simulink model "WESDem_SetPoint"  (R2016b)
settings: configuration reference "CodeGenConfigSet" (kept outside this file)
values from neighbouring files (symbols this model uses):
  EISGov_st3valid_C = Calibration.Parameter    [init_WESDem_SetPoint.m]
  WESDem_dnAcc0_C = Calibration.Parameter    [init_WESDem_SetPoint.m]
  WESDem_dnAcc1_C = Calibration.Parameter    [init_WESDem_SetPoint.m]
  WESDem_dnAcc3_C = Calibration.Parameter    [init_WESDem_SetPoint.m]
  WESDem_dnDecn0_C = Calibration.Parameter    [init_WESDem_SetPoint.m]
  WESDem_dnDecn1_C = Calibration.Parameter    [init_WESDem_SetPoint.m]
  WESDem_dnDecn2_C = Calibration.Parameter    [init_WESDem_SetPoint.m]
  WESDem_nDelta_C = Calibration.Parameter    [init_WESDem_SetPoint.m]
  WESDem_nMin0_C = Calibration.Parameter    [init_WESDem_SetPoint.m]
  WESDem_nMin1_C = Calibration.Parameter    [init_WESDem_SetPoint.m]
  WESDem_nMin2_C = Calibration.Parameter    [init_WESDem_SetPoint.m]
  WESDem_nMin3_C = Calibration.Parameter    [init_WESDem_SetPoint.m]
  WESDem_nMode0_C = Calibration.Parameter    [init_WESDem_SetPoint.m]
  WESDem_nMode1_C = Calibration.Parameter    [init_WESDem_SetPoint.m]
  WESDem_nMode2_C = Calibration.Parameter    [init_WESDem_SetPoint.m]
  WESDem_nMode3_C = Calibration.Parameter    [init_WESDem_SetPoint.m]
  WESDem_nSetPHi0_C = Calibration.Parameter    [init_WESDem_SetPoint.m]
  WESDem_nSetPHi1_C = Calibration.Parameter    [init_WESDem_SetPoint.m]
  WESDem_nSetPHi2_C = Calibration.Parameter    [init_WESDem_SetPoint.m]
  WESDem_nSetPHi3_C = Calibration.Parameter    [init_WESDem_SetPoint.m]
  WESDem_nTipStp_C = Calibration.Parameter    [init_WESDem_SetPoint.m]
  WESDem_rAPPThresFrzI_C = Calibration.Parameter    [init_WESDem_SetPoint.m]
  WESDem_SetPLoTipInRmpSlopeNeg_C = Calibration.Parameter    [init_WESDem_SetPoint.m]
  WESDem_SetPLoTipInRmpSlopePos_C = Calibration.Parameter    [init_WESDem_SetPoint.m]
  WESDem_stASDrfInit_C = Calibration.Parameter    [init_WESDem_SetPoint.m]
  WESDem_stCurr_C = Calibration.Parameter    [init_WESDem_SetPoint.m]
  WESDem_stCurrvalid_C = Calibration.Parameter    [init_WESDem_SetPoint.m]
  WESDem_stMskFrzRls_C = Calibration.Parameter    [init_WESDem_SetPoint.m]
  WESDem_swtTrqHiSel_C = Calibration.Parameter    [init_WESDem_SetPoint.m]
  WESDem_swtTrqLoSel_C = Calibration.Parameter    [init_WESDem_SetPoint.m]
  WESDem_tiPT1_C = Calibration.Parameter    [init_WESDem_SetPoint.m]
  WESDem_tiTrqHiPT1_C = Calibration.Parameter    [init_WESDem_SetPoint.m]
  WESDem_tiTrqLoPT1_C = Calibration.Parameter    [init_WESDem_SetPoint.m]
undefined symbols (not defined in the file or in its folder): CruiseCtl_State_conv, Switch_conv, WESDem_SetPoint_DT, WESDem_State_conv
libraries: CXLib x23, simulink x15
(part 2 of 2)

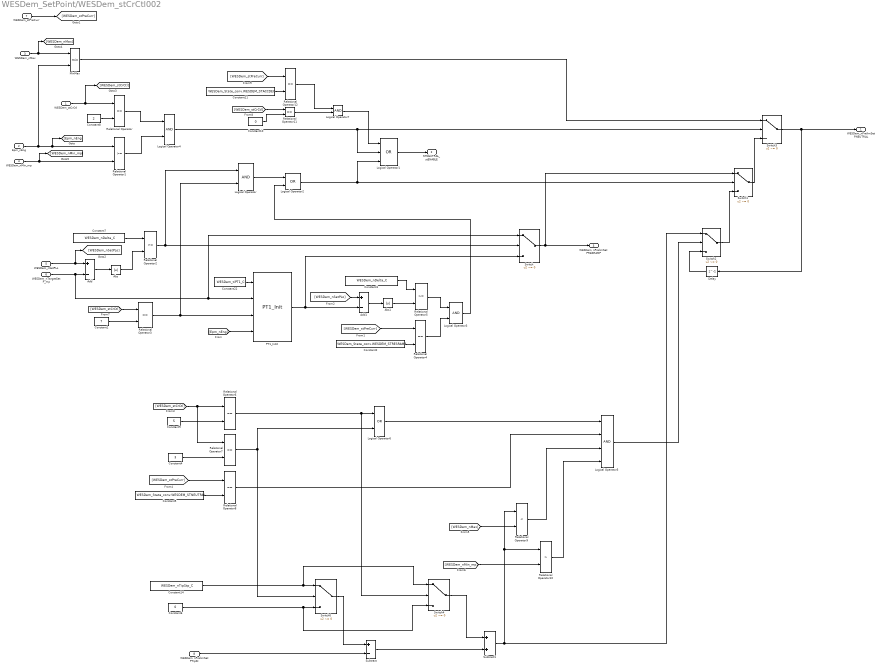
== system WESDem_SetPoint/WESDem_stCrCtl002  ==
  WESDem_stCrCtl : Inport  Description=State control of the working engine speed demand  OutMin=0  OutMax=65535  OutDataTypeStr=State_uint16
  Epm_nEng : Inport  Tag=rpm  Description=Engine speed  Port=2  OutMin=0  OutMax=6000  OutDataTypeStr=EngSpeed_rpm
  WESDem_nMax : Inport  Tag=rpm  Description=Engine speed  Port=3  OutMin=0  OutMax=6000  OutDataTypeStr=EngSpeed_rpm
  WESDem_nMin_mp : Inport  Tag=rpm  Description=Engine speed  Port=4  OutMin=0  OutMax=6000  OutDataTypeStr=EngSpeed_rpm
  WESDem_nSetPLo : Inport  Port=5
  WESDem_nTargetSetP_mp : Inport  Port=6
  WESDem_stPreCurr : Inport  Description=State control of the working engine speed demand  Port=7  OutDataTypeStr=Enum: WESDem_State_conv
  WESDem_nPrelimSetPTipSt : Inport  Port=8
  Abs : Abs
  Abs1 : Abs
  Add : Sum  Inputs=+-
  Add1 : Sum  Inputs=+-
  Constant1 : Constant  Value=7  OutDataTypeStr=Inherit: Inherit via back propagation
  Constant10 : Constant  Value=0  OutDataTypeStr=Inherit: Inherit via back propagation
  Constant11 : Constant  Value=WESDem_State_conv.WESDEM_STACCDEC  OutDataTypeStr=Inherit: Inherit via back propagation
  Constant14 : Constant  Value=WESDem_nTipStp_C
  Constant2 : Constant  Value=WESDem_State_conv.WESDEM_STRESRAMP  OutDataTypeStr=Inherit: Inherit via back propagation
  Constant22 : Constant  Value=WESDem_tiPT1_C
  Constant3 : Constant  Value=WESDem_nDelta_C
  Constant4 : Constant  Value=3  OutDataTypeStr=Inherit: Inherit via back propagation
  Constant5 : Constant  Value=WESDem_State_conv.WESDEM_STNEUTRAL  OutDataTypeStr=Inherit: Inherit via back propagation
  Constant6 : Constant  Value=0  OutDataTypeStr=Inherit: Inherit via back propagation
  Constant7 : Constant  Value=WESDem_nDelta_C
  Constant8 : Constant  Value=2  OutDataTypeStr=Inherit: Inherit via back propagation
  Constant9 : Constant  Value=5  OutDataTypeStr=Inherit: Inherit via back propagation
  Delay : Delay  DelayLength=1  InitialCondition=0
  Logical Operator{,3..4,7} (4 alike) : Logic  AllPortsSameDT=off  OutDataTypeStr=boolean
  Logical Operator1 : Logic  Operator=OR  Inputs=3  AllPortsSameDT=off  OutDataTypeStr=boolean
  Logical Operator2 : Logic  Operator=OR  AllPortsSameDT=off  OutDataTypeStr=boolean
  Logical Operator5 : Logic  Inputs=4  AllPortsSameDT=off  OutDataTypeStr=boolean
  Logical Operator6 : Logic  Operator=OR  AllPortsSameDT=off  OutDataTypeStr=boolean
  MinMax : MinMax  Inputs=2
  PT1_Init2 : CXLib/PT1_Init
  Relational Operator{,3..4,8,11..12} (6 alike) : RelationalOperator  Operator===  OutDataTypeStr=boolean  RndMeth=Simplest
  Relational Operator1 : RelationalOperator  OutDataTypeStr=boolean  RndMeth=Simplest
  Relational Operator10 : RelationalOperator  Operator=>  OutDataTypeStr=boolean  RndMeth=Simplest
  Relational Operator2 : RelationalOperator  OutDataTypeStr=boolean  RndMeth=Simplest
  Relational Operator5 : RelationalOperator  OutDataTypeStr=boolean  RndMeth=Simplest
  Relational Operator6 : RelationalOperator  Operator===  OutDataTypeStr=boolean  RndMeth=Simplest  InputSameDT=on
  Relational Operator7 : RelationalOperator  Operator===  OutDataTypeStr=boolean  RndMeth=Simplest  InputSameDT=on
  Relational Operator9 : RelationalOperator  Operator=<  OutDataTypeStr=boolean  RndMeth=Simplest
  Subtract : Sum  Inputs=+-
  Subtract1 : Sum
  Switch{,1..4,6} (6 alike) : Switch  Criteria=u2 ~= 0
  WESDem_nPrelimSetPNEUTRAL : Outport  Tag=rpm  Description=maximum engine speed in selected mode  OutMin=0  OutMax=6000  OutDataTypeStr=EngSpeed_rpm
  STNEUTRAL_stENABLE : Outport  Port=2
  WESDem_nPrelimSetPRESRAMP : Outport  Port=3
  wires:
  WESDem_stCrCtl/1 -> Relational Operator/1, [WESDem_stCrCtl]
  Constant8/1 -> Relational Operator/2
  Epm_nEng/1 -> MinMax/2, Relational Operator1/1, [Epm_nEng]
  WESDem_nMin_mp/1 -> Relational Operator1/2, [WESDem_nMin_mp]
  Relational Operator/1 -> Logical Operator4/1
  Relational Operator1/1 -> Logical Operator4/2
  WESDem_nMax/1 -> MinMax/1, [WESDem_nMax]
  MinMax/1 -> Switch3/1
  Logical Operator4/1 -> Logical Operator1/2, Switch3/2
  Switch3/1 -> Delay/1, WESDem_nPrelimSetPNEUTRAL/1
  Abs/1 -> Relational Operator2/2
  Constant7/1 -> Relational Operator2/1
  WESDem_nSetPLo/1 -> [WESDem_nSetPLo], Add/1
  Add/1 -> Abs/1
  WESDem_nTargetSetP_mp/1 -> Switch/1, PT1_Init2/2, Add/2
  Constant1/1 -> Relational Operator3/2
  Relational Operator2/1 -> Logical Operator/1, Switch/2
  Logical Operator1/1 -> STNEUTRAL_stENABLE/1
  WESDem_stPreCurr/1 -> [WESDem_stPreCurr]
  PT1_Init2/1 -> Switch/3, Add1/2
  Constant22/1 -> PT1_Init2/1
  Relational Operator3/1 -> Logical Operator/2, PT1_Init2/3
  [Epm_nEng] -> PT1_Init2/4
  Switch1/1 -> Switch3/3
  Switch/1 -> WESDem_nPrelimSetPRESRAMP/1, Switch1/1
  Logical Operator/1 -> Logical Operator2/1
  Constant2/1 -> Relational Operator4/2
  [WESDem_stPreCurr] -> Relational Operator4/1
  Add1/1 -> Abs1/1
  [WESDem_nSetPLo] -> Add1/1
  Constant3/1 -> Relational Operator5/1
  Abs1/1 -> Relational Operator5/2
  Relational Operator5/1 -> Logical Operator3/1
  Relational Operator4/1 -> Logical Operator3/2
  Logical Operator3/1 -> Logical Operator2/2
  Logical Operator2/1 -> Logical Operator1/3, Switch1/2
  Delay/1 -> Switch2/3
  [WESDem_stCrCtl] -> Relational Operator7/1, Relational Operator6/1
  Constant9/1 -> Relational Operator6/2
  Constant4/1 -> Relational Operator7/2
  Relational Operator7/1 -> Switch6/2, Logical Operator6/2
  Relational Operator6/1 -> Switch4/2, Logical Operator6/1
  [WESDem_stPreCurr] -> Relational Operator8/1
  Constant5/1 -> Relational Operator8/2
  Logical Operator6/1 -> Logical Operator5/1
  Relational Operator8/1 -> Logical Operator5/2
  [WESDem_nMax] -> Relational Operator9/2
  Relational Operator9/1 -> Logical Operator5/3
  [WESDem_nMin_mp] -> Relational Operator10/2
  Constant6/1 -> Switch4/3, Switch6/3
  Constant14/1 -> Switch4/1, Switch6/1
  WESDem_nPrelimSetPTipSt/1 -> Subtract/2
  Switch6/1 -> Subtract/1
  Switch4/1 -> Subtract1/1
  Subtract/1 -> Subtract1/2
  Relational Operator10/1 -> Logical Operator5/4
  Subtract1/1 -> Switch2/1, Relational Operator10/1, Relational Operator9/1
  Logical Operator5/1 -> Switch2/2
  Switch2/1 -> Switch1/3
  [WESDem_stCrCtl] -> Relational Operator3/1
  [WESDem_stCrCtl] -> Relational Operator11/1
  Constant10/1 -> Relational Operator11/2
  Relational Operator11/1 -> Logical Operator7/2
  Constant11/1 -> Relational Operator12/2
  [WESDem_stPreCurr] -> Relational Operator12/1
  Relational Operator12/1 -> Logical Operator7/1
  Logical Operator7/1 -> Logical Operator1/1

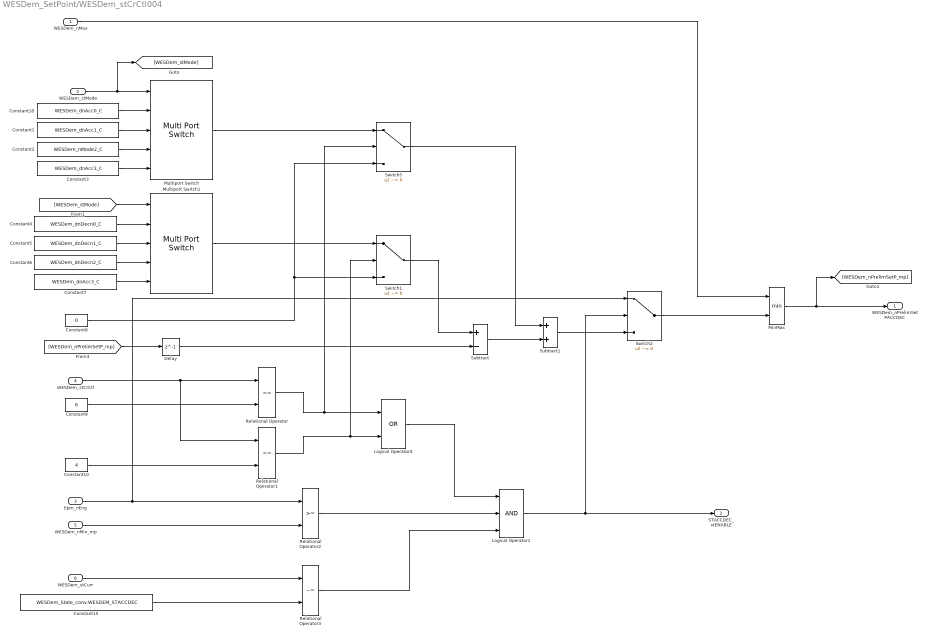
== system WESDem_SetPoint/WESDem_stCrCtl004 ==
  WESDem_nMax : Inport  Tag=rpm  Description=Working engine speed setpoint through start button  OutMin=0  OutMax=6000  OutDataTypeStr=EngSpeed_rpm
  WESDem_stMode : Inport  Description=Operating mode of the working engine speed demand  Port=2  OutMin=0  OutMax=255  OutDataTypeStr=State_uint8
  Epm_nEng : Inport  Tag=rpm  Description=Engine speed  Port=3  OutMin=0  OutMax=6000  OutDataTypeStr=EngSpeed_rpm
  WESDem_stCrCtl : Inport  Description=State control of the working engine speed demand  Port=4  OutMin=0  OutMax=65535  OutDataTypeStr=State_uint16
  WESDem_nMin_mp : Inport  Port=5
  WESDem_stCurr : Inport  Port=6
  Constant1 : Constant  Value=WESDem_dnAcc1_C
  Constant10 : Constant  Value=4
  Constant15 : Constant  Value=WESDem_State_conv.WESDEM_STACCDEC  OutDataTypeStr=Inherit: Inherit via back propagation
  Constant18 : Constant  Value=WESDem_dnAcc0_C
  Constant2 : Constant  Value=WESDem_nMode2_C
  Constant3 : Constant  Value=WESDem_dnAcc3_C
  Constant4 : Constant  Value=WESDem_dnDecn0_C
  Constant5 : Constant  Value=WESDem_dnDecn1_C
  Constant6 : Constant  Value=WESDem_dnDecn2_C
  Constant7 : Constant  Value=WESDem_dnAcc3_C
  Constant8 : Constant  Value=0  OutDataTypeStr=Inherit: Inherit via back propagation
  Constant9 : Constant  Value=6
  Delay : Delay  DelayLength=1  InitialCondition=0
  Logical Operator1 : Logic  Inputs=3  AllPortsSameDT=off  OutDataTypeStr=boolean
  Logical Operator4 : Logic  Operator=OR  AllPortsSameDT=off  OutDataTypeStr=boolean
  MinMax : MinMax  Inputs=2
  Multiport Switch : MultiPortSwitch  DataPortOrder=Zero-based contiguous  Inputs=4
  Multiport Switch1 : MultiPortSwitch  DataPortOrder=Zero-based contiguous  Inputs=4
  Relational Operator : RelationalOperator  Operator===  OutDataTypeStr=boolean  RndMeth=Simplest
  Relational Operator1 : RelationalOperator  Operator===  OutDataTypeStr=boolean  RndMeth=Simplest
  Relational Operator2 : RelationalOperator  OutDataTypeStr=boolean  RndMeth=Simplest
  Relational Operator3 : RelationalOperator  Operator=~=  OutDataTypeStr=boolean  RndMeth=Simplest
  Subtract : Sum  Inputs=+-
  Subtract1 : Sum
  Switch1 : Switch  Criteria=u2 ~= 0
  Switch2 : Switch  Criteria=u2 ~= 0
  Switch5 : Switch  Criteria=u2 ~= 0
  WESDem_nPrelimSetPACCDEC : Outport  Tag=rpm  Description=maximum engine speed in selected mode  OutMin=0  OutMax=6000  OutDataTypeStr=EngSpeed_rpm
  STACCDEC_stENABLE : Outport  Port=2
  wires:
  WESDem_stMode/1 -> [WESDem_stMode], Multiport Switch/1
  Constant1/1 -> Multiport Switch/3
  Constant2/1 -> Multiport Switch/4
  Constant3/1 -> Multiport Switch/5
  Constant18/1 -> Multiport Switch/2
  Constant4/1 -> Multiport Switch1/2
  Constant5/1 -> Multiport Switch1/3
  Constant6/1 -> Multiport Switch1/4
  Constant7/1 -> Multiport Switch1/5
  Multiport Switch/1 -> Switch5/1
  Multiport Switch1/1 -> Switch1/1
  Constant8/1 -> Switch1/3, Switch5/3
  Switch1/1 -> Subtract/1
  Delay/1 -> Subtract/2
  Switch5/1 -> Subtract1/1
  Subtract/1 -> Subtract1/2
  Subtract1/1 -> Switch2/3
  WESDem_stCrCtl/1 -> Relational Operator1/1, Relational Operator/1
  Constant9/1 -> Relational Operator/2
  Constant10/1 -> Relational Operator1/2
  Relational Operator/1 -> Switch5/2, Logical Operator4/1
  Relational Operator1/1 -> Switch1/2, Logical Operator4/2
  Epm_nEng/1 -> Switch2/1, Relational Operator2/1
  [WESDem_stMode] -> Multiport Switch1/1
  Constant15/1 -> Relational Operator3/2
  Relational Operator3/1 -> Logical Operator1/3
  Relational Operator2/1 -> Logical Operator1/2
  Logical Operator4/1 -> Logical Operator1/1
  Logical Operator1/1 -> Switch2/2, STACCDEC_stENABLE/1
  Switch2/1 -> MinMax/2
  WESDem_nMax/1 -> MinMax/1
  MinMax/1 -> [WESDem_nPrelimSetP_mp], WESDem_nPrelimSetPACCDEC/1
  [WESDem_nPrelimSetP_mp] -> Delay/1
  WESDem_nMin_mp/1 -> Relational Operator2/2
  WESDem_stCurr/1 -> Relational Operator3/1

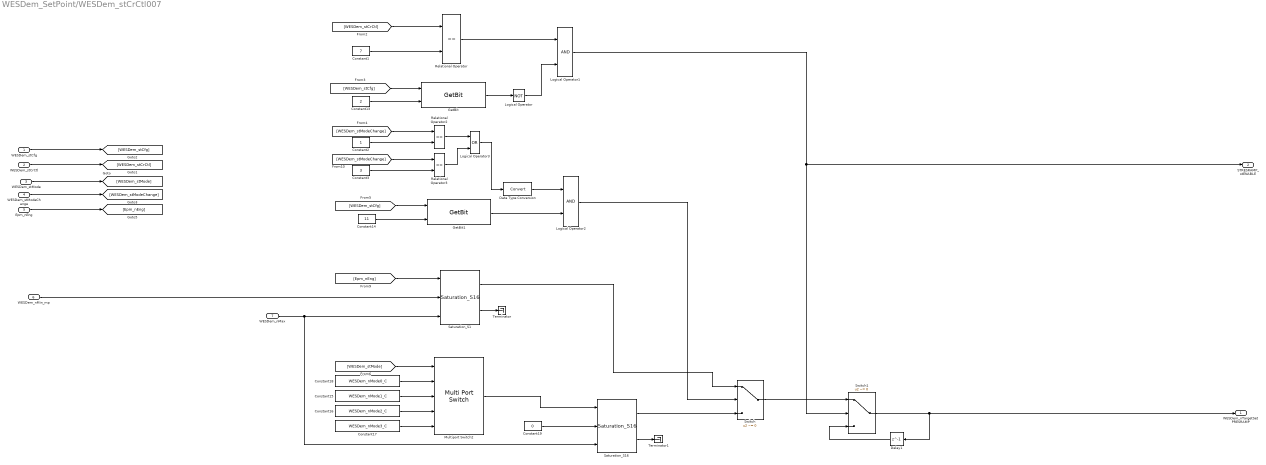
== system WESDem_SetPoint/WESDem_stCrCtl007 ==
  WESDem_stCfg : Inport  Description=Configuration of the actual operating mode  OutMin=0  OutMax=65535  OutDataTypeStr=State_uint16
  WESDem_stCrCtl : Inport  Description=State control of the working engine speed demand  Port=2  OutMin=0  OutMax=65535  OutDataTypeStr=State_uint16
  WESDem_stMode : Inport  Description=Operating mode of the working engine speed demand  Port=3  OutMin=0  OutMax=255  OutDataTypeStr=State_uint8
  WESDem_stModeChange : Inport  Description=Operating mode change of the working engine speed demand  Port=4  OutMin=0  OutMax=255  OutDataTypeStr=State_uint8
  Epm_nEng : Inport  Tag=rpm  Description=Engine speed  Port=5  OutMin=0  OutMax=6000  OutDataTypeStr=EngSpeed_rpm
  WESDem_nMin_mp : Inport  Port=6
  WESDem_nMax : Inport  Port=7
  Constant1 : Constant  Value=7  OutDataTypeStr=Inherit: Inherit via back propagation
  Constant13 : Constant  Value=2  OutDataTypeStr=Inherit: Inherit via back propagation
  Constant14 : Constant  Value=11  OutDataTypeStr=Inherit: Inherit via back propagation
  Constant15 : Constant  Value=WESDem_nMode1_C
  Constant16 : Constant  Value=WESDem_nMode2_C
  Constant17 : Constant  Value=WESDem_nMode3_C
  Constant18 : Constant  Value=WESDem_nMode0_C
  Constant19 : Constant  Value=0  OutDataTypeStr=Inherit: Inherit via back propagation
  Constant2 : Constant  OutDataTypeStr=Inherit: Inherit via back propagation
  Constant3 : Constant  Value=3  OutDataTypeStr=Inherit: Inherit via back propagation
  Data Type Conversion : DataTypeConversion
  Delay1 : Delay  DelayLength=1  InitialCondition=0
  GetBit : CXLib/GetBit  dataTypeString=uint16  dataLength=0
      settings: AttributesFormatString=Get bit from %<dataTypeString>
  GetBit1 : CXLib/GetBit  dataTypeString=uint16  dataLength=0
      settings: AttributesFormatString=Get bit from %<dataTypeString>
  Logical Operator : Logic  Operator=NOT  AllPortsSameDT=off  OutDataTypeStr=boolean
  Logical Operator1 : Logic  AllPortsSameDT=off  OutDataTypeStr=boolean
  Logical Operator2 : Logic  AllPortsSameDT=off  OutDataTypeStr=boolean
  Logical Operator3 : Logic  Operator=OR  AllPortsSameDT=off  OutDataTypeStr=boolean
  Multiport Switch2 : MultiPortSwitch  DataPortOrder=Zero-based contiguous  Inputs=4
  Relational Operator : RelationalOperator  Operator===  OutDataTypeStr=boolean  RndMeth=Simplest
  Relational Operator2 : RelationalOperator  Operator===  OutDataTypeStr=boolean  RndMeth=Simplest
  Relational Operator3 : RelationalOperator  Operator===  OutDataTypeStr=boolean  RndMeth=Simplest
  Saturation_S1 : CXLib/Saturation_S16
  Saturation_S16 : CXLib/Saturation_S16
  Switch : Switch  Criteria=u2 ~= 0
  Switch1 : Switch  Criteria=u2 ~= 0
  Terminator : Terminator
  Terminator1 : Terminator
  WESDem_nTargetSetPRESRAMP : Outport  Description=Status of the working engine Speed Control  OutMin=0  OutMax=6000  OutDataTypeStr=EngSpeed_rpm
  STRESRAMP_stENABLE : Outport  Port=2
  wires:
  Delay1/1 -> Switch1/3
  WESDem_stCrCtl/1 -> [WESDem_stCrCtl]
  WESDem_stMode/1 -> [WESDem_stMode]
  Relational Operator/1 -> Logical Operator1/1
  [WESDem_stCfg] -> GetBit1/1
  Epm_nEng/1 -> [Epm_nEng]
  Saturation_S1/1 -> Switch/1
  Constant14/1 -> GetBit1/2
  [Epm_nEng] -> Saturation_S1/1
  WESDem_stModeChange/1 -> [WESDem_stModeChange]
  Logical Operator/1 -> Logical Operator1/2
  Saturation_S16/1 -> Switch/3
  Multiport Switch2/1 -> Saturation_S16/1
  WESDem_nMax/1 -> Saturation_S16/3, Saturation_S1/3
  [WESDem_stMode] -> Multiport Switch2/1
  GetBit1/1 -> Logical Operator2/2
  Constant15/1 -> Multiport Switch2/3
  Logical Operator2/1 -> Switch/2
  Constant19/1 -> Saturation_S16/2
  WESDem_stCfg/1 -> [WESDem_stCfg]
  [WESDem_stCfg] -> GetBit/1
  Constant13/1 -> GetBit/2
  Constant1/1 -> Relational Operator/2
  Constant18/1 -> Multiport Switch2/2
  GetBit/1 -> Logical Operator/1
  Constant16/1 -> Multiport Switch2/4
  [WESDem_stCrCtl] -> Relational Operator/1
  Constant17/1 -> Multiport Switch2/5
  Saturation_S16/2 -> Terminator1/1
  Switch/1 -> Switch1/1
  Logical Operator1/1 -> STRESRAMP_stENABLE/1, Switch1/2
  Saturation_S1/2 -> Terminator/1
  Switch1/1 -> Delay1/1, WESDem_nTargetSetPRESRAMP/1
  Data Type Conversion/1 -> Logical Operator2/1
  [WESDem_stModeChange] -> Relational Operator2/1
  Constant2/1 -> Relational Operator2/2
  [WESDem_stModeChange] -> Relational Operator3/1
  Constant3/1 -> Relational Operator3/2
  Relational Operator2/1 -> Logical Operator3/1
  Relational Operator3/1 -> Logical Operator3/2
  Logical Operator3/1 -> Data Type Conversion/1
  WESDem_nMin_mp/1 -> Saturation_S1/2

== stateflow chart WESDem_SetPoint/EISGov initialization/Chart ==
  state WESDEM_STNOINIT
    entry:WESDem_stEISGovInit_mp = 0;
  state WESDEM_STONINIT
    entry:WESDem_stEISGovInit_mp = 2;
  state WESDEM_STOFFINIT
    entry:WESDem_stEISGovInit_mp = 1;
  (default) -> WESDEM_STNOINIT
  WESDEM_STNOINIT -> WESDEM_STONINIT [order 2] : [NoInitToOnInit_st ==1]
  WESDEM_STNOINIT -> WESDEM_STOFFINIT [order 1] : [NoInitToOffInit_st == 1]
  WESDEM_STONINIT -> WESDEM_STNOINIT : [OnInitToNoInit_st == 1]
  WESDEM_STOFFINIT -> WESDEM_STNOINIT : [OffInitToNoInit_st ==1]
  data: NoInitToOnInit_st input; NoInitToOffInit_st input; OffInitToNoInit_st input; OnInitToNoInit_st input; WESDem_stEISGovInit_mp output
